simulink model "lengthy_simulation"  (R2015a)
settings: Solver=ode45  StartTime=0.0  StopTime=10.0  RelTol=1e-3
libraries: simulink x11
settings Model: Creator=shafiul  LastModifiedBy=shafiul

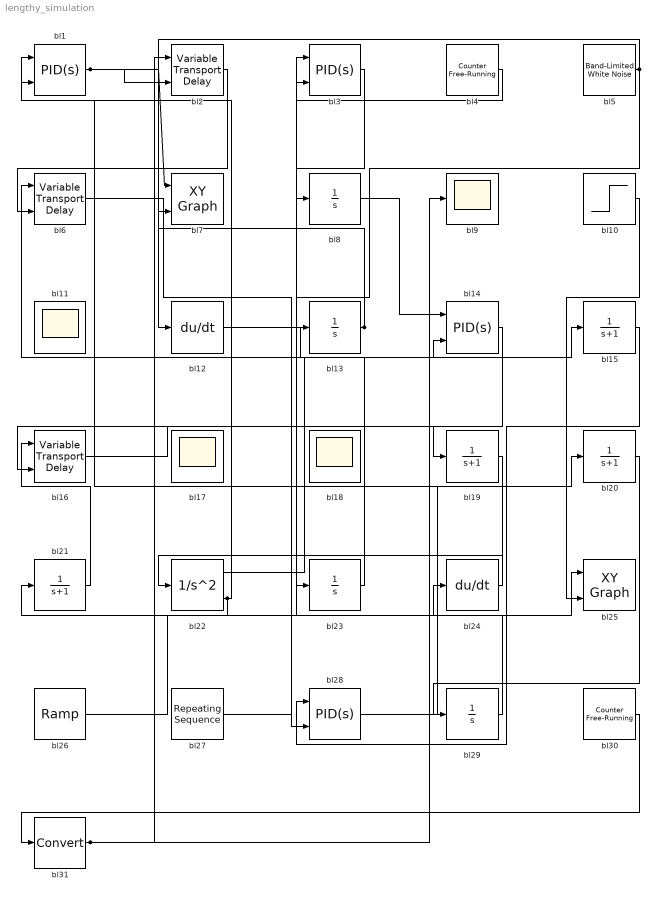
== system lengthy_simulation ==
  bl{1,3,14,28} (4 alike) : simulink/Continuous/PID Controller (2DOF)  Controller=PID  TimeDomain=Continuous-time  SampleTime=-1  IntegratorMethod=Forward Euler  FilterMethod=Forward Euler  Form=Parallel  UseFilter=on  ControllerParametersSource=internal  P=1  I=1  D=0  N=100  b=1  c=1  InitialConditionSource=internal  InitialConditionForIntegrator=0  InitialConditionForFilter=0  ExternalReset=none  LimitOutput=off  UpperSaturationLimit=inf  LowerSaturationLimit=-inf  LinearizeAsGain=on  AntiWindupMode=none  Kb=1  TrackingMode=off  Kt=1  PParamMin=[]  PParamMax=[]  IParamMin=[]  IParamMax=[]  DParamMin=[]  DParamMax=[]  NParamMin=[]  NParamMax=[]  bParamMin=[]  bParamMax=[]  cParamMin=[]  cParamMax=[]  KbParamMin=[]  KbParamMax=[]  KtParamMin=[]  KtParamMax=[]  POutMin=[]  POutMax=[]  IOutMin=[]  IOutMax=[]  DOutMin=[]  DOutMax=[]  NOutMin=[]  NOutMax=[]  bOutMin=[]  bOutMax=[]  cOutMin=[]  cOutMax=[]  KbOutMin=[]  KbOutMax=[]  KtOutMin=[]  KtOutMax=[]  IntegratorOutMin=[]  IntegratorOutMax=[]  FilterOutMin=[]  FilterOutMax=[]  SumOutMin=[]  SumOutMax=[]  Sum1OutMin=[]  Sum1OutMax=[]  Sum2OutMin=[]  Sum2OutMax=[]  Sum3OutMin=[]  Sum3OutMax=[]  SumI1OutMin=[]  SumI1OutMax=[]  SumI2OutMin=[]  SumI2OutMax=[]  SumI3OutMin=[]  SumI3OutMax=[]  SumDOutMin=[]  SumDOutMax=[]  SaturationOutMin=[]  SaturationOutMax=[]  IntegratorContinuousStateAttributes=''  IntegratorStateMustResolveToSignalObject=off  IntegratorRTWStateStorageClass=Auto  FilterContinuousStateAttributes=''  FilterStateMustResolveToSignalObject=off  FilterRTWStateStorageClass=Auto  DifferentiatorICPrevScaledInput=0  DifferentiatorOutMin=[]  DifferentiatorOutMax=[]
  bl10 : Step  After=21  SampleTime=0
  bl{9,11,17..18} (4 alike) : Scope
      bl11 settings: Floating=on
      bl17 settings: Floating=on
      bl18 settings: Floating=on
  bl12 : Derivative
  bl{8,13,23,29} (4 alike) : Integrator  LimitOutput=on  UpperSaturationLimit=1  LowerSaturationLimit=0
  bl{15,19..21} (4 alike) : TransferFcn  Denominator=[1 1]
  bl16 : VariableTransportDelay  MaximumDelay=10  InitialOutput=811
  bl2 : VariableTransportDelay  MaximumDelay=10  InitialOutput=777
  bl22 : SecondOrderIntegrator
  bl24 : Derivative
  bl25 : simulink/Sinks/XY Graph  xmin=-1  xmax=1  ymin=-1  ymax=1  st=-1
  bl26 : simulink/Sources/Ramp  slope=1  start=0  X0=0
  bl27 : simulink/Sources/Repeating Sequence  rep_seq_t=[0 2]  rep_seq_y=[0 2]
  bl30 : simulink/Sources/Counter Free-Running  NumBits=16  tsamp=-1
  bl31 : DataTypeConversion
  bl4 : simulink/Sources/Counter Free-Running  NumBits=16  tsamp=-1
  bl5 : simulink/Sources/Band-Limited White Noise  Cov=[0.1]  Ts=0.1  seed=[23341]
  bl6 : VariableTransportDelay  MaximumDelay=10  InitialOutput=164
  bl7 : simulink/Sinks/XY Graph  xmin=-1  xmax=1  ymin=-1  ymax=1  st=-1
  wires:
  bl28/1 -> bl20/1
  bl22/1 -> bl15/1
  bl29/1 -> bl3/1
  bl21/1 -> bl16/1
  bl24/1 -> bl1/1
  bl3/1 -> bl23/1
  bl8/1 -> bl14/1
  bl12/1 -> bl14/2
  bl5/1 -> bl12/1, bl13/1
  bl1/1 -> bl7/1, bl2/2
  bl20/1 -> bl28/1
  bl6/1 -> bl28/2
  bl26/1 -> bl25/1
  bl14/1 -> bl16/2
  bl23/1 -> bl6/1
  bl2/1 -> bl6/2
  bl19/1 -> bl22/1
  bl22/2 -> bl21/1, bl1/2
  bl13/1 -> bl8/1, bl7/2
  bl10/1 -> bl25/2
  bl27/1 -> bl24/1
  bl16/1 -> bl19/1
  bl30/1 -> bl31/1
  bl4/1 -> bl3/2
  bl15/1 -> bl29/1
  bl31/1 -> bl2/1, bl9/1
